simulink library "fast_library"  (Simulink 8.1)
settings: Solver=ode45  StartTime=0.0  StopTime=10.0  RelTol=1e-3
libraries: xbsIndex_r4 x439, casper_library_misc x3, xps_library x2
(part 1 of 3)
settings Model: Creator=zhuyan  LastModifiedBy=zhuyan

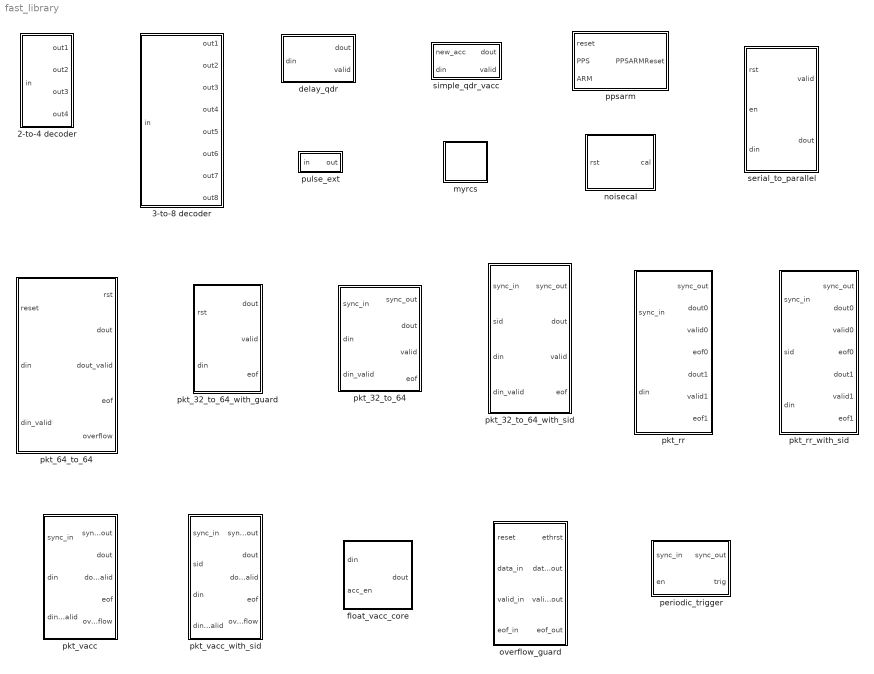
== system fast_library ==
  2-to-4 decoder : Subsystem  mask(decoder_2_4){}
      mask help: 2 to 4 decoder
  3-to-8 decoder : Subsystem  mask(decoder_3_8){}
      mask help: 3 to 8 decoder
  delay_qdr : Subsystem  mask(delay_qdr){DelayLen=1022, qdr_slot=qdr1}
      mask prompts: DelayLen "Delay Length (even number >=14):"; qdr_slot "QDR Slot:"
      mask init:
      | set_param([gcb, '/qdr'], 'which_qdr', qdr_slot);
      mask TypeOptions qdr_slot: qdr0 | qdr1 | qdr2 | qdr3
  float_vacc_core : Subsystem  mask(float_vacc_core){veclen=16, arith_type=1, conv_latency=3, add_latency=2, bram_latency=2, mux_latency=1}
      mask prompts: veclen "Vector Length"; arith_type "Arithmetic Type (0=Unsigned, 1=Signed)"; conv_latency "Convert Lantency"; add_latency "Add Latency"; bram_latency "BRAM Latency"; mux_latency "Mux Latency"
      mask help:
      | Currently only Signed arithmetic supported
      | acc_en = 0 --> Load a vector (start a new accumulation)
      | acc_en = 1 --> Accumulate
      mask init:
      | float_vacc_core_init(gcb, ...
      |     'veclen', veclen, ...
      |     'arith_type', arith_type, ...
      |     'conv_latency', conv_latency, ...
      |     'add_latency', add_latency, ...
      |     'bram_latency', bram_latency, ...
      |     'mux_latency', mux_latency);
  myrcs : Subsystem  mask(myrcs){proj_id=MYID}
      mask prompts: proj_id "Project ID:"
      mask help:
      | Revision control block.
      |
      | proj_id - exact 4 characters filled by user.
      | timestamp - seconds from unix epoch.
      | version - high 16 bits are major and low 16 bits are minor.
      |
      | The timestamp and version are taken from model properties.
      mask init:
      | blk = gcb();
      | sys = bdroot();
      | 
      | if length(proj_id) ~= 4
      |     error('Project ID must be exact 4 characters');
      | end
      | 
      | set_param(blk, 'LinkStatus', 'inactive')
      | 
      | rcs_id = proj_id(1)*256^3 + proj_id(2)*256^2 + proj_id(3)*256 + proj_id(4);
      | set_param([blk '/rcs_id'], 'const', num2str(rcs_id));
      | 
      | unix_epoch = datenum(1970, 1, 1, 0, 0, 0);
      | mdate = datenum(get_param(sys, 'LastModifiedDate'), 'ddd mmm dd HH:MM:SS yyyy');
      | unix_time = round((mdate - unix_epoch) * 24*60*60);
      | set_param([blk '/rcs_timestamp'], 'const', num2str(unix_time));
      | 
      | vers = sscanf(get_param(sys, 'ModelVersion'), '%d.%d');
      | rcs_ver = num2str(vers(1)*65536 + vers(2));
      | set_param([blk '/rcs_ver'], 'const', rcs_ver);
      mask Display: fprintf(proj_id);
  noisecal : Subsystem  mask(noisecal){}
      mask help:
      | Square wave to control external noise source.
      |
      | delay - number of clocks before the noise on signal after reset+latency
      | on - number of clocks in on state
      | off -number of clocks in off state
      |
      | sequence:
      | reset->delay->on->off->on->off->...
      mask Display:
      | port_label('input', 1, 'rst');
      | port_label('output', 1, 'cal');
      | disp('z^{-5}','texmode','on');
  overflow_guard : Subsystem  mask(overflow_guard){}
      mask help: Overflow gardian to ten_Gbe_v2 block
  periodic_trigger : Subsystem  mask(periodic_trigger){period=3}
  pkt_32_to_64 : Subsystem  mask(pkt_32_to_64){nbits=10}
      mask prompts: nbits "Packet Size in input length (2^?) :"
      mask help: packetizer 32-bits wide input into 64-bits wide packets and insert a 64-bit serial number at the packet head.
      mask init:
      | dstr = sprintf('packet length: %d bytes', 2^nbits * 4 + 8);
      | set_param(gcb, 'AttributesFormatString', dstr);
      settings: AttributesFormatString=packet length: 4104 bytes
      mask Display:
      | port_label('input', 1, 'sync_in');
      | port_label('input', 2, 'din');
      | port_label('input', 3, 'din_valid');
      | port_label('output', 1, 'sync_out');
      | port_label('output', 2, 'dout');
      | port_label('output', 3, 'valid');
      | port_label('output', 4, 'eof');
      | color('black');disp('z^{-3}','texmode','on');
  pkt_32_to_64_with_guard : Subsystem  mask(pkt_32_to_64_with_guard){nbits=10}
      mask prompts: nbits "Packet Size in input length (2^?) :"
      mask help:
      | valid data output 4 cycles later than reset signal.
      | serial number start from 1 (instead of 0) after reset signal.
      | Issue 10GbE block a reset signal before reset this block
      mask Display:
      | port_label('input', 1, 'rst');
      | port_label('input', 2, 'din');
      | port_label('output', 1, 'dout');
      | port_label('output', 2, 'valid');
      | port_label('output', 3, 'eof');
      | color('black');disp('z^{-4}','texmode','on');
      | fprintf('\n\n\n%dB', 2^nbits * 4 + 8);
  pkt_32_to_64_with_sid : Subsystem  mask(pkt_32_to_64_with_sid){nbits=10}
      mask prompts: nbits "Packet Size in input length (2^?) :"
      mask help: packetizer 32-bit wide input into 64-bit wide packets and insert a 64-bit header which consist of one 8-bit sid and one 56-bit serial number before sending out packet data.
      mask init:
      | dstr = sprintf('packet length: %d bytes', 2^nbits * 4 + 8);
      | set_param(gcb, 'AttributesFormatString', dstr);
      settings: AttributesFormatString=packet length: 4104 bytes
      mask Display:
      | port_label('input', 1, 'sync_in');
      | port_label('input', 2, 'sid');
      | port_label('input', 3, 'din');
      | port_label('input', 4, 'din_valid');
      | port_label('output', 1, 'sync_out');
      | port_label('output', 2, 'dout');
      | port_label('output', 3, 'valid');
      | port_label('output', 4, 'eof');
      | color('black');disp('z^{-3}','texmode','on');
  pkt_64_to_64 : Subsystem  mask{pktlen=1024, idlecycles=640, fifo_depth=2K}
      mask prompts: pktlen "Packet length in INPUT word (64bit):"; idlecycles "Idle cycles between packet:"; fifo_depth "FIFO depth (in 64bit word):"
      mask TypeOptions fifo_depth: 16 | 32 | 64 | 128 | 256 | 512 | 1K | 2K | 4K | 8K | 16K | 32K | 64K | 128K | 256K | 512K | 1M | 2M | 4M
  pkt_rr : Subsystem  mask(pkt_rr){nbits=9}
      mask prompts: nbits "Packet Size: (2^?)"
      mask help:
      | Split continous 64 bit input stream into packets and add one 64 bit serial number at each packet head.
      |
      | The output packets are placed into 2 output ports round robin, to match 2 10GbE yellow block.
      |
      | The packet size is counted in number of 64 bit (8 bytes) input word, the recommended packet size is 9 (4096 bytes).
  pkt_rr_with_sid : Subsystem  mask(pkt_rr_with_sid){nbits=9}
      mask prompts: nbits "Packet Size: (2^?)"
      mask help:
      | Split continous 64 bit input stream into packets and add one 64 bit serial number at each packet head.
      |
      | The output packets are placed into 2 output ports round robin, to match 2 10GbE yellow block.
      |
      | The packet size is counted in number of 64 bit (8 bytes) input word, the recommended packet size is 9 (4096 bytes).
  pkt_vacc : Subsystem  mask(pkt_vacc){spec_bits=8, pkt_bits=8, fifo_depth=16}
      mask prompts: spec_bits "Spectrum Size (2^?) in 64-bit word:"; pkt_bits "Packet Size (2^?):"; fifo_depth "FIFO Depth:"
      mask help:
      | For packetize bulk vacc output.
      |
      | 1. Split spectrum longer than 2^9 words (4k bytes) into 2^9 words packets.
      | 2. Leave spectrum shorter than 2^9 words as one single packet.
      | 3. Add a 64-bit serial number for each packet.
      mask init:
      | if spec_bits < pkt_bits
      |     error('Packet size should be equal or smaller than Spectrum size!');
      | elseif pkt_bits == spec_bits
      |     fifo_depth = '16';
      | elseif spec_bits > 20
      |     error('Spectrum size too large! should < 20');
      | else
      |     if spec_bits > 10
      |         fifo_depth = [num2str(2^(spec_bits - 11)) 'K'];
      |     else
      |         fifo_depth = num2str(2^(spec_bits - 1));
      |     end
      | end
      | 
      | % msgbox(fifo_depth);
      | %set_param([gcb '/FIFO'], 'depth', fifo_depth);
      | 
      | set_param(gcb, 'fifo_depth', fifo_depth);
  pkt_vacc_with_sid : Subsystem  mask(pkt_vacc_with_sid){spec_bits=8, pkt_bits=8, fifo_depth=16}
      mask prompts: spec_bits "Spectrum Size (2^?) in 64-bit word:"; pkt_bits "Packet Size (2^?):"; fifo_depth "FIFO Depth:"
      mask help:
      | For packetize bulk vacc output.
      |
      | 1. Split spectrum longer than 2^9 words (4k bytes) into 2^9 words packets.
      | 2. Leave spectrum shorter than 2^9 words as one single packet.
      | 3. Add a 64-bit serial number for each packet.
      mask init: same as fast_library/pkt_vacc
  ppsarm : Subsystem  mask(ppsarm){}
      mask help: PPS-ARM machanism
  pulse_ext : Subsystem  mask(pulse_ext){pulse_len=2}
      mask prompts: pulse_len "Length of Pulse"
      mask help: Extends a boolean signal to be high for the specified number of clocks after the last high input.
      mask init:
      | bits = ceil(log2(pulse_len+1));
      mask Help: eval('xlWeb(''http://casper.berkeley.edu/wiki/Pulse_ext'')')
  serial_to_parallel : Subsystem  mask(serial_to_parallel){n_elems=4}
      mask prompts: n_elems "Number of Parallel Elements:"
      mask init:
      | serial_to_parallel_init(gcb, ...
      |     'n_elems', n_elems)
  simple_qdr_vacc : Subsystem  mask(simple_qdr_vacc){vec_len=94, arith_type=Signed, n_bits=32, bin_pt=5, qdr_slot=qdr0}
      mask prompts: vec_len "Vector length (even number):"; arith_type "Output type:"; n_bits "Bit width (output):"; bin_pt "Binary point (output):"; qdr_slot "QDR slot:"
      mask help: It will output accumulated value from the 2nd new_acc
      mask init:
      | simple_qdr_vacc_init(gcb, ...
      |     'vec_len', vec_len, ...
      |     'arith_type', arith_type, ...
      |     'n_bits', n_bits, ...
      |     'bin_pt', bin_pt, ...
      |     'qdr_slot', qdr_slot);
      mask TypeOptions arith_type: Signed | Unsigned
      mask TypeOptions qdr_slot: qdr0 | qdr1 | qdr2 | qdr3

== system fast_library/2-to-4 decoder ==
  in : Inport
  Inverter : xbsIndex_r4/Inverter  en=off  latency=0  dbl_ovrd=off  block_type=inv
  Inverter1 : xbsIndex_r4/Inverter  en=off  latency=0  dbl_ovrd=off  block_type=inv
  Logical{,1..3} (4 alike) : xbsIndex_r4/Logical  logical_function=AND  inputs=2  en=off  latency=0  precision=Full  arith_type=Unsigned  n_bits=16  bin_pt=0  align_bp=on  dbl_ovrd=off  block_type=logical
  high bit : xbsIndex_r4/Slice  nbits=1  boolean_output=off  mode=Upper Bit Location + Width  bit1=0  base1=MSB of Input  bit0=0  base0=LSB of Input  dbl_ovrd=off  block_type=slice
  low bit : xbsIndex_r4/Slice  nbits=1  boolean_output=off  mode=Lower Bit Location + Width  bit1=0  base1=MSB of Input  bit0=0  base0=LSB of Input  dbl_ovrd=off  block_type=slice
  out1 : Outport
  out2 : Outport  Port=2
  out3 : Outport  Port=3
  out4 : Outport  Port=4
  wires:
  Logical2/1 -> out3/1
  Logical1/1 -> out2/1
  Logical/1 -> out1/1
  Inverter/1 -> Logical2/2, Logical/1
  high bit/1 -> Logical3/2, Logical2/1, Inverter1/1
  low bit/1 -> Logical3/1, Logical1/1, Inverter/1
  Logical3/1 -> out4/1
  Inverter1/1 -> Logical1/2, Logical/2
  in/1 -> low bit/1, high bit/1

== system fast_library/3-to-8 decoder ==
  in : Inport
  2-to-4 decoder : Subsystem
  2-to-4 decoder1 : Subsystem
  Inverter : xbsIndex_r4/Inverter  en=off  latency=0  dbl_ovrd=off  block_type=inv
  Slice : xbsIndex_r4/Slice  nbits=1  boolean_output=off  mode=Lower Bit Location + Width  bit1=0  base1=MSB of Input  bit0=1  base0=LSB of Input  dbl_ovrd=off  block_type=slice
  Slice1 : xbsIndex_r4/Slice  nbits=1  boolean_output=off  mode=Lower Bit Location + Width  bit1=0  base1=MSB of Input  bit0=0  base0=LSB of Input  dbl_ovrd=off  block_type=slice
  Slice2 : xbsIndex_r4/Slice  nbits=1  boolean_output=off  mode=Lower Bit Location + Width  bit1=0  base1=MSB of Input  bit0=2  base0=LSB of Input  dbl_ovrd=off  block_type=slice
  out1 : Outport
  out2 : Outport  Port=2
  out3 : Outport  Port=3
  out4 : Outport  Port=4
  out5 : Outport  Port=5
  out6 : Outport  Port=6
  out7 : Outport  Port=7
  out8 : Outport  Port=8
  wires:
  Slice2/1 -> 2-to-4 decoder1/3(EN), Inverter/1
  Slice1/1 -> 2-to-4 decoder1/1(A), 2-to-4 decoder/1(A)
  2-to-4 decoder1/4(D3) -> out8/1
  2-to-4 decoder/3(D2) -> out3/1
  2-to-4 decoder1/3(D2) -> out7/1
  2-to-4 decoder1/1(D0) -> out5/1
  2-to-4 decoder/4(D3) -> out4/1
  2-to-4 decoder/2(D1) -> out2/1
  2-to-4 decoder/1(D0) -> out1/1
  2-to-4 decoder1/2(D1) -> out6/1
  in/1 -> Slice1/1, Slice2/1, Slice/1
  Inverter/1 -> 2-to-4 decoder/3(EN)
  Slice/1 -> 2-to-4 decoder1/2(B), 2-to-4 decoder/2(B)

== system fast_library/delay_qdr ==
  din : Inport
  Constant3 : xbsIndex_r4/Constant  const=15  gui_display_data_type=Fixed-point  arith_type=Unsigned  n_bits=4  bin_pt=0  preci_type=Single  exp_width=8  frac_width=24  explicit_period=off  period=1  equ=P=C  opselect=C  inp2=PCIN>>17  opr=+  inp1=P  carry=CIN  dbl_ovrd=off  block_type=constant
  Constant4 : xbsIndex_r4/Constant  const=DelayLen-10-4  gui_display_data_type=Fixed-point  arith_type=Unsigned  n_bits=nextpow2(DelayLen)  bin_pt=0  preci_type=Single  exp_width=8  frac_width=24  explicit_period=on  period=1  equ=P=C  opselect=C  inp2=PCIN>>17  opr=+  inp1=P  carry=CIN  dbl_ovrd=off  block_type=constant
  Convert : xbsIndex_r4/Convert  gui_display_data_type=Fixed-point  arith_type=Unsigned  n_bits=36  bin_pt=0  float_type=Single  exp_bits=8  fraction_bits=24  quantization=Truncate  overflow=Wrap  en=off  latency=0  dbl_ovrd=off  pipeline=off  block_type=convert
      settings: block_version=11.4
  Delay : xbsIndex_r4/Delay  rst=off  infoeditControl=Selection of Reset will increase slice count due to use of real FFs and instead of SRLs  en=off  latency=1  dbl_ovrd=off  reg_retiming=off  block_type=delay
  Delay1 : xbsIndex_r4/Delay  rst=off  infoeditControl=Selection of Reset will increase slice count due to use of real FFs and instead of SRLs  en=off  latency=1  dbl_ovrd=off  reg_retiming=off  block_type=delay
  Delay2 : xbsIndex_r4/Delay  rst=off  infoeditControl=Selection of Reset will increase slice count due to use of real FFs and instead of SRLs  en=off  latency=1  dbl_ovrd=off  reg_retiming=off  block_type=delay
  Gateway Out{1..6} (6 alike) : xbsIndex_r4/Gateway Out  inherit_from_input=off  hdl_port=on  timing_constraint=None  locs_specified=off  LOCs={}  UseAsDAC=off  DACChannel='1'  block_type=gatewayout
  Inverter2 : xbsIndex_r4/Inverter  en=off  latency=0  dbl_ovrd=off  block_type=inv
  Mux3 : xbsIndex_r4/Mux  inputs=2  en=off  latency=0  precision=Full  arith_type="Signed  (2's comp)"  n_bits=8  bin_pt=2  quantization=Truncate  overflow=Wrap  dbl_ovrd=off  block_type=mux
      settings: xl_area=[0, 0, 0, 0, 0, 0, 0]
  Reinterpret : xbsIndex_r4/Reinterpret  force_arith_type=on  arith_type=Unsigned  force_bin_pt=on  bin_pt=0  block_type=reinterpret
  Relational : xbsIndex_r4/Relational  mode=a=b  en=off  latency=0  dbl_ovrd=off  block_type=relational
  Scope : Scope  NumInputPorts=6
      settings: YMin=-5~-5~-5~-5~-5~-5  YMax=5~5~5~5~5~5  SaveName=Scope
  Slice1 : xbsIndex_r4/Slice  nbits=1  boolean_output=off  mode=Two Bit Locations  bit1=0  base1=MSB of Input  bit0=1  base0=LSB of Input  dbl_ovrd=off  block_type=slice
  Slice2 : xbsIndex_r4/Slice  nbits=1  boolean_output=off  mode=Two Bit Locations  bit1=0  base1=MSB of Input  bit0=1  base0=LSB of Input  dbl_ovrd=off  block_type=slice
  Terminator : Terminator
  Terminator1 : Terminator
  Terminator2 : Terminator
  qdr : xps_library/qdr  Tag=xps:qdr  which_qdr=qdr1  qdr_awidth=12  use_sniffer=off
  rd/wr : xbsIndex_r4/Counter  cnt_type=Free Running  cnt_to=Inf  operation=Up  start_count=1  cnt_by_val=1  arith_type=Unsigned  n_bits=1  bin_pt=0  load_pin=off  rst=off  en=off  explicit_period=on  period=1  dbl_ovrd=off  use_behavioral_HDL=off  implementation=Fabric  block_type=counter
  rd_addr : xbsIndex_r4/Counter  cnt_type=Count Limited  cnt_to=DelayLen-1  operation=Up  start_count=0  cnt_by_val=1  arith_type=Unsigned  n_bits=nextpow2(DelayLen)  bin_pt=0  load_pin=off  rst=on  en=off  explicit_period=on  period=1  dbl_ovrd=off  use_behavioral_HDL=off  implementation=Fabric  use_rpm=off  block_type=counter
      settings: xl_area=[0, 0, 0, 0, 0, 0, 0]
  wr_addr : xbsIndex_r4/Counter  cnt_type=Count Limited  cnt_to=DelayLen-1  operation=Up  start_count=0  cnt_by_val=1  arith_type=Unsigned  n_bits=nextpow2(DelayLen)  bin_pt=0  load_pin=off  rst=off  en=off  explicit_period=on  period=1  dbl_ovrd=off  use_behavioral_HDL=off  implementation=Fabric  use_rpm=off  block_type=counter
      settings: xl_area=[0, 0, 0, 0, 0, 0, 0]
  dout : Outport
  valid : Outport  Port=2
  wires:
  Slice2/1 -> Mux3/3
  qdr/5 -> Terminator2/1
  Constant4/1 -> Relational/2
  Mux3/1 -> Gateway Out2/1, qdr/4
  Convert/1 -> Gateway Out3/1, qdr/5
  qdr/3 -> Terminator/1
  rd_addr/1 -> Slice1/1
  wr_addr/1 -> Relational/1, Slice2/1
  Delay/1 -> rd_addr/1
  Constant3/1 -> qdr/3
  qdr/4 -> Terminator1/1
  Relational/1 -> Delay/1
  Slice1/1 -> Mux3/2
  qdr/2 -> Delay2/1
  qdr/1 -> Delay1/1
  Gateway Out6/1 -> Scope/1
  Gateway Out1/1 -> Scope/2
  Gateway Out2/1 -> Scope/3
  Gateway Out3/1 -> Scope/4
  Gateway Out4/1 -> Scope/5
  Gateway Out5/1 -> Scope/6
  rd/wr/1 -> Gateway Out1/1, qdr/2, Inverter2/1, Mux3/1
  Inverter2/1 -> Gateway Out6/1, qdr/1
  Delay1/1 -> Gateway Out5/1, dout/1
  Delay2/1 -> Gateway Out4/1, valid/1
  din/1 -> Reinterpret/1
  Reinterpret/1 -> Convert/1

== system fast_library/float_vacc_core ==
  note: This BRAM and counter is exactly what is inside the green
      | Delay BRAM block. The functionality was extracted to avoid
      | library issues.
  din : Inport
  acc_en : Inport  Port=2
  Adder : xbsIndex_r4/AddSub  mode=Addition  use_carryin=off  use_carryout=off  en=off  latency=2  precision=Full  arith_type="Signed  (2's comp)"  n_bits=32  bin_pt=7  quantization=Truncate  overflow=Wrap  dbl_ovrd=off  use_behavioral_HDL=on  hw_selection=Fabric  pipelined=on  use_rpm=on  block_type=addsub
      settings: xl_area=[0, 0, 0, 0, 0, 0, 0]  block_version=10.1.2
  BRAM : xbsIndex_r4/Single Port RAM  depth=16  initVector=0  distributed_mem=Block RAM  write_mode=Read Before Write  rst=off  init_reg=0  en=off  latency=2  dbl_ovrd=off  optimize=Area  block_type=spram
      settings: xl_area=[0, 0, 0, 0, 0, 0, 0]  block_version=10.1.2
  Constant : xbsIndex_r4/Constant  const=0  gui_display_data_type=Floating-point  arith_type=Floating-point  n_bits=1  bin_pt=0  preci_type=Single  exp_width=8  frac_width=24  explicit_period=on  period=1  equ=P=C  opselect=C  inp2=PCIN>>17  opr=+  inp1=P  carry=CIN  dbl_ovrd=off  block_type=constant
      settings: block_version=10.1.2
  Constant2 : xbsIndex_r4/Constant  const=1  gui_display_data_type=Fixed-point  arith_type=Boolean  n_bits=1  bin_pt=0  preci_type=Single  exp_width=8  frac_width=24  explicit_period=on  period=1  equ=P=C  opselect=C  inp2=PCIN>>17  opr=+  inp1=P  carry=CIN  dbl_ovrd=off  block_type=constant
      settings: block_version=10.1.2
  Convert : xbsIndex_r4/Convert  gui_display_data_type=Floating-point  arith_type=Floating-point  n_bits=16  bin_pt=14  float_type=Single  exp_bits=8  fraction_bits=24  quantization=Truncate  overflow=Wrap  en=off  latency=3  dbl_ovrd=off  pipeline=on  block_type=convert
  Counter : xbsIndex_r4/Counter  cnt_type=Count Limited  cnt_to=7  operation=Up  start_count=0  cnt_by_val=1  arith_type=Unsigned  n_bits=4  bin_pt=0  load_pin=off  rst=off  en=off  explicit_period=off  period=1  dbl_ovrd=off  use_behavioral_HDL=off  implementation=Fabric  use_rpm=off  block_type=counter
      settings: xl_area=[0, 0, 0, 0, 0, 0, 0]  block_version=10.1.2
  Delay : xbsIndex_r4/Delay  rst=off  infoeditControl=Selection of Reset will increase slice count due to use of real FFs and instead of SRLs  en=off  latency=3  dbl_ovrd=off  reg_retiming=off  block_type=delay
  Delay1 : xbsIndex_r4/Delay  rst=off  infoeditControl=Selection of Reset will increase slice count due to use of real FFs and instead of SRLs  en=off  latency=3  dbl_ovrd=off  reg_retiming=off  block_type=delay
  Mux : xbsIndex_r4/Mux  inputs=2  en=off  latency=1  precision=Full  arith_type="Signed  (2's comp)"  n_bits=8  bin_pt=2  quantization=Truncate  overflow=Wrap  dbl_ovrd=off  block_type=mux
      settings: xl_area=[0, 0, 0, 0, 0, 0, 0]  block_version=10.1.2
  dout : Outport
  wires:
  acc_en/1 -> Delay/1
  Constant/1 -> Mux/2
  din/1 -> Convert/1
  Adder/1 -> dout/1, BRAM/2
  Counter/1 -> BRAM/1
  Constant2/1 -> BRAM/3
  Convert/1 -> Adder/1
  Delay/1 -> Mux/1
  Mux/1 -> Adder/2
  BRAM/1 -> Delay1/1
  Delay1/1 -> Mux/3

== system fast_library/myrcs ==
  id : Subsystem  Tag=xps:sw_reg  AncestorBlock=xps_library/software register  mask(swreg){io_dir=To Processor, io_delay=0, sample_period=1, names=reg, bitwidths=32, bin_pts=0, arith_types=0, sim_port=off, show_format=on}
      mask prompts: io_dir "I/O direction"; io_delay "I/O delay"; sample_period "Sample period"; names "Bitfield names [msb...lsb]"; bitwidths "Bitfield widths"; bin_pts "Bitfield binary pts"; arith_types "Bitfield types, ufix=0, fix=1, bool=2"; sim_port "Provide sim input/output?"; show_format "Print format string?"
      mask help: A 32-bit software-accessible register. Can be divided into bitfields of varying widths and types using the fields in the block mask.
      mask init:
      | swreg_init(gcb)
      settings: AttributesFormatString=1output:uf32.0
      mask TypeOptions io_dir: To Processor | From Processor
      mask Callback io_dir:
      | mask_enables = get_param(gcb, 'MaskEnables');
      | mask_names = get_param(gcb, 'MaskNames');
      | if strcmp(get_param(gcb, 'io_dir'), 'To Processor'),
      |     mask_enables{ismember(mask_names, 'sample_period')} = 'off';
      | else
      |     mask_enables{ismember(mask_names, 'sample_period')} = 'on';
      | end
      | set_param(gcb, 'MaskEnables', mask_enables);
  rcs_id : xbsIndex_r4/Constant  const=1297697092  gui_display_data_type=Fixed-point  arith_type=Unsigned  n_bits=32  bin_pt=0  preci_type=Single  exp_width=8  frac_width=24  explicit_period=on  period=1  equ=P=C  opselect=C  inp2=PCIN>>17  opr=+  inp1=P  carry=CIN  dbl_ovrd=off  block_type=constant
  rcs_timestamp : xbsIndex_r4/Constant  const=1550549974  gui_display_data_type=Fixed-point  arith_type=Unsigned  n_bits=32  bin_pt=0  preci_type=Single  exp_width=8  frac_width=24  explicit_period=on  period=1  equ=P=C  opselect=C  inp2=PCIN>>17  opr=+  inp1=P  carry=CIN  dbl_ovrd=off  block_type=constant
  rcs_ver : xbsIndex_r4/Constant  const=65582  gui_display_data_type=Fixed-point  arith_type=Unsigned  n_bits=32  bin_pt=0  preci_type=Single  exp_width=8  frac_width=24  explicit_period=on  period=1  equ=P=C  opselect=C  inp2=PCIN>>17  opr=+  inp1=P  carry=CIN  dbl_ovrd=off  block_type=constant
  timestamp : Subsystem  Tag=xps:sw_reg  AncestorBlock=xps_library/software register  mask(swreg){io_dir=To Processor, io_delay=0, sample_period=1, names=reg, bitwidths=32, bin_pts=0, arith_types=0, sim_port=off, show_format=on}
      mask prompts: io_dir "I/O direction"; io_delay "I/O delay"; sample_period "Sample period"; names "Bitfield names [msb...lsb]"; bitwidths "Bitfield widths"; bin_pts "Bitfield binary pts"; arith_types "Bitfield types, ufix=0, fix=1, bool=2"; sim_port "Provide sim input/output?"; show_format "Print format string?"
      mask help: A 32-bit software-accessible register. Can be divided into bitfields of varying widths and types using the fields in the block mask.
      mask init:
      | swreg_init(gcb)
      settings: AttributesFormatString=1output:uf32.0
      mask TypeOptions io_dir: To Processor | From Processor
      mask Callback io_dir:
      | mask_enables = get_param(gcb, 'MaskEnables');
      | mask_names = get_param(gcb, 'MaskNames');
      | if strcmp(get_param(gcb, 'io_dir'), 'To Processor'),
      |     mask_enables{ismember(mask_names, 'sample_period')} = 'off';
      | else
      |     mask_enables{ismember(mask_names, 'sample_period')} = 'on';
      | end
      | set_param(gcb, 'MaskEnables', mask_enables);
  ver : Subsystem  Tag=xps:sw_reg  AncestorBlock=xps_library/software register  mask(swreg){io_dir=To Processor, io_delay=0, sample_period=1, names=reg, bitwidths=32, bin_pts=0, arith_types=0, sim_port=off, show_format=on}
      mask prompts: io_dir "I/O direction"; io_delay "I/O delay"; sample_period "Sample period"; names "Bitfield names [msb...lsb]"; bitwidths "Bitfield widths"; bin_pts "Bitfield binary pts"; arith_types "Bitfield types, ufix=0, fix=1, bool=2"; sim_port "Provide sim input/output?"; show_format "Print format string?"
      mask help: A 32-bit software-accessible register. Can be divided into bitfields of varying widths and types using the fields in the block mask.
      mask init:
      | swreg_init(gcb)
      settings: AttributesFormatString=1output:uf32.0
      mask TypeOptions io_dir: To Processor | From Processor
      mask Callback io_dir:
      | mask_enables = get_param(gcb, 'MaskEnables');
      | mask_names = get_param(gcb, 'MaskNames');
      | if strcmp(get_param(gcb, 'io_dir'), 'To Processor'),
      |     mask_enables{ismember(mask_names, 'sample_period')} = 'off';
      | else
      |     mask_enables{ismember(mask_names, 'sample_period')} = 'on';
      | end
      | set_param(gcb, 'MaskEnables', mask_enables);
  wires:
  rcs_id/1 -> id/1(out_reg)
  rcs_ver/1 -> ver/1(out_reg)
  rcs_timestamp/1 -> timestamp/1(out_reg)

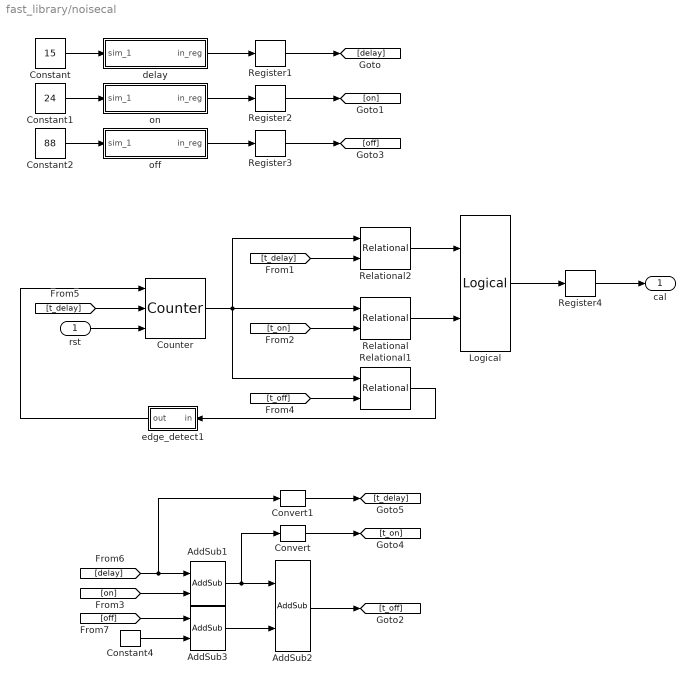
== system fast_library/noisecal ==
  rst : Inport
  AddSub1 : xbsIndex_r4/AddSub  mode=Addition  use_carryin=off  use_carryout=off  en=off  latency=2  precision=Full  arith_type=Unsigned  n_bits=32  bin_pt=0  quantization=Truncate  overflow=Wrap  dbl_ovrd=off  use_behavioral_HDL=on  hw_selection=Fabric  pipelined=off  block_type=addsub
  AddSub2 : xbsIndex_r4/AddSub  mode=Addition  use_carryin=off  use_carryout=off  en=off  latency=2  precision=Full  arith_type=Unsigned  n_bits=32  bin_pt=0  quantization=Truncate  overflow=Wrap  dbl_ovrd=off  use_behavioral_HDL=on  hw_selection=Fabric  pipelined=off  block_type=addsub
  AddSub3 : xbsIndex_r4/AddSub  mode=Subtraction  use_carryin=off  use_carryout=off  en=off  latency=2  precision=User Defined  arith_type=Unsigned  n_bits=33  bin_pt=0  quantization=Truncate  overflow=Wrap  dbl_ovrd=off  use_behavioral_HDL=on  hw_selection=Fabric  pipelined=off  block_type=addsub
  Constant : Constant  Value=15
  Constant1 : Constant  Value=24
  Constant2 : Constant  Value=88
  Constant4 : xbsIndex_r4/Constant  const=3  gui_display_data_type=Fixed-point  arith_type=Unsigned  n_bits=2  bin_pt=0  preci_type=Single  exp_width=8  frac_width=24  explicit_period=on  period=1  equ=P=C  opselect=C  inp2=PCIN>>17  opr=+  inp1=P  carry=CIN  dbl_ovrd=off  block_type=constant
  Convert : xbsIndex_r4/Convert  gui_display_data_type=Fixed-point  arith_type=Unsigned  n_bits=34  bin_pt=0  float_type=Single  exp_bits=8  fraction_bits=24  quantization=Truncate  overflow=Wrap  en=off  latency=2  dbl_ovrd=off  pipeline=off  block_type=convert
  Convert1 : xbsIndex_r4/Convert  gui_display_data_type=Fixed-point  arith_type=Unsigned  n_bits=34  bin_pt=0  float_type=Single  exp_bits=8  fraction_bits=24  quantization=Truncate  overflow=Wrap  en=off  latency=4  dbl_ovrd=off  pipeline=off  block_type=convert
  Counter : xbsIndex_r4/Counter  cnt_type=Free Running  cnt_to=Inf  operation=Up  start_count=0  cnt_by_val=1  arith_type=Unsigned  n_bits=34  bin_pt=0  load_pin=on  rst=on  en=off  explicit_period=on  period=1  dbl_ovrd=off  use_behavioral_HDL=on  implementation=Fabric  block_type=counter
  Logical : xbsIndex_r4/Logical  logical_function=XOR  inputs=2  en=off  latency=1  precision=Full  arith_type=Unsigned  n_bits=16  bin_pt=0  align_bp=on  dbl_ovrd=off  block_type=logical
  Register{1..4} (4 alike) : xbsIndex_r4/Register  init=0  rst=off  en=off  dbl_ovrd=off  block_type=register
  Relational : xbsIndex_r4/Relational  mode=a<b  en=off  latency=2  dbl_ovrd=off  block_type=relational
  Relational1 : xbsIndex_r4/Relational  mode=a<b  en=off  latency=2  dbl_ovrd=off  block_type=relational
  Relational2 : xbsIndex_r4/Relational  mode=a<b  en=off  latency=2  dbl_ovrd=off  block_type=relational
  delay : Subsystem  Tag=xps:sw_reg  AncestorBlock=xps_library/software register  mask(swreg){io_dir=From Processor, io_delay=0, sample_period=1, names=reg, bitwidths=32, bin_pts=0, arith_types=0, sim_port=on, show_format=off}
      mask prompts: io_dir "I/O direction"; io_delay "I/O delay"; sample_period "Sample period"; names "Bitfield names [msb...lsb]"; bitwidths "Bitfield widths"; bin_pts "Bitfield binary pts"; arith_types "Bitfield types, ufix=0, fix=1, bool=2"; sim_port "Provide sim input/output?"; show_format "Print format string?"
      mask help: A 32-bit software-accessible register. Can be divided into bitfields of varying widths and types using the fields in the block mask.
      mask init:
      | swreg_init(gcb)
      settings: AttributesFormatString=1input
      mask TypeOptions io_dir: To Processor | From Processor
      mask Callback io_dir:
      | mask_enables = get_param(gcb, 'MaskEnables');
      | mask_names = get_param(gcb, 'MaskNames');
      | if strcmp(get_param(gcb, 'io_dir'), 'To Processor'),
      |     mask_enables{ismember(mask_names, 'sample_period')} = 'off';
      | else
      |     mask_enables{ismember(mask_names, 'sample_period')} = 'on';
      | end
      | set_param(gcb, 'MaskEnables', mask_enables);
  edge_detect1 : Subsystem  AncestorBlock=casper_library_misc/edge_detect  mask(edge_detect){edge=Falling, polarity=Active High, x_in=[0 0.08 0.08 0.16 0.16 0.24 0.24 0.32 0.32 0.4], y_in=[-1 -1  1  1  1  1  1  1  1  1], x_out=[0.6 0.68 0.68 0.76 0.76 0.84 0.84 0.92 0.92 1], y_out=[-1 -1  1  1 -1 -1 -1 -1 -1 -1]}
      mask prompts: edge "Edge Type"; polarity "Output Polarity"; x_in "Input X Positions"; y_in "Input Y Positions"; x_out "Output X Positions"; y_out "Output Y Positions"
      mask help: Output is active for one-cycle after each edge of the specified type (i.e. rising, falling or both).
      mask init:
      | edge_detect_init(gcb,...
      |     'edge',edge,...
      |     'polarity',polarity,...
      |     'x_in',x_in,...
      |     'x_out',x_out,...
      |     'y_in',y_in,...
      |     'y_out',y_out);
      | 
      | x_in_num=str2num(getfield(getfield(get_param(gcb,'UserData'),'parameters'),'x_in'));
      | x_out_num=str2num(getfield(getfield(get_param(gcb,'UserData'),'parameters'),'x_out'));
      | y_in_num=str2num(getfield(getfield(get_param(gcb,'UserData'),'parameters'),'y_in'));
      | y_out_num=str2num(getfield(getfield(get_param(gcb,'UserData'),'parameters'),'y_out'));
      settings: AttributesFormatString=|
      | falling edges
      | active high
      mask Help: Output is active for one-cycle after each edge of the specified type (i.e. rising, falling, or both).  Latency is zero.
      mask TypeOptions edge: Rising | Falling | Both
      mask TypeOptions polarity: Active High | Active Low
      mask Display:
      | plot(x_in_num,0.5+y_in_num*0.2);
      | plot(x_out_num,0.5+y_out_num*0.2);
  off : Subsystem  Tag=xps:sw_reg  AncestorBlock=xps_library/software register  mask(swreg){io_dir=From Processor, io_delay=0, sample_period=1, names=reg, bitwidths=32, bin_pts=0, arith_types=0, sim_port=on, show_format=off}
      mask prompts: io_dir "I/O direction"; io_delay "I/O delay"; sample_period "Sample period"; names "Bitfield names [msb...lsb]"; bitwidths "Bitfield widths"; bin_pts "Bitfield binary pts"; arith_types "Bitfield types, ufix=0, fix=1, bool=2"; sim_port "Provide sim input/output?"; show_format "Print format string?"
      mask help: A 32-bit software-accessible register. Can be divided into bitfields of varying widths and types using the fields in the block mask.
      mask init:
      | swreg_init(gcb)
      settings: AttributesFormatString=1input
      mask TypeOptions io_dir: To Processor | From Processor
      mask Callback io_dir:
      | mask_enables = get_param(gcb, 'MaskEnables');
      | mask_names = get_param(gcb, 'MaskNames');
      | if strcmp(get_param(gcb, 'io_dir'), 'To Processor'),
      |     mask_enables{ismember(mask_names, 'sample_period')} = 'off';
      | else
      |     mask_enables{ismember(mask_names, 'sample_period')} = 'on';
      | end
      | set_param(gcb, 'MaskEnables', mask_enables);
  on : Subsystem  Tag=xps:sw_reg  AncestorBlock=xps_library/software register  mask(swreg){io_dir=From Processor, io_delay=0, sample_period=1, names=reg, bitwidths=32, bin_pts=0, arith_types=0, sim_port=on, show_format=off}
      mask prompts: io_dir "I/O direction"; io_delay "I/O delay"; sample_period "Sample period"; names "Bitfield names [msb...lsb]"; bitwidths "Bitfield widths"; bin_pts "Bitfield binary pts"; arith_types "Bitfield types, ufix=0, fix=1, bool=2"; sim_port "Provide sim input/output?"; show_format "Print format string?"
      mask help: A 32-bit software-accessible register. Can be divided into bitfields of varying widths and types using the fields in the block mask.
      mask init:
      | swreg_init(gcb)
      settings: AttributesFormatString=1input
      mask TypeOptions io_dir: To Processor | From Processor
      mask Callback io_dir:
      | mask_enables = get_param(gcb, 'MaskEnables');
      | mask_names = get_param(gcb, 'MaskNames');
      | if strcmp(get_param(gcb, 'io_dir'), 'To Processor'),
      |     mask_enables{ismember(mask_names, 'sample_period')} = 'off';
      | else
      |     mask_enables{ismember(mask_names, 'sample_period')} = 'on';
      | end
      | set_param(gcb, 'MaskEnables', mask_enables);
  cal : Outport
  wires:
  Convert1/1 -> [t_delay]
  Convert/1 -> [t_on]
  [t_off] -> Relational1/2
  AddSub2/1 -> [t_off]
  AddSub3/1 -> AddSub2/2
  Constant4/1 -> AddSub3/2
  [off] -> AddSub3/1
  AddSub1/1 -> AddSub2/1, Convert/1
  [on] -> AddSub1/2
  [delay] -> AddSub1/1, Convert1/1
  Register4/1 -> cal/1
  Relational1/1 -> edge_detect1/1(in)
  delay/1(in_reg) -> Register1/1
  Constant2/1 -> off/1(sim_1)
  Constant1/1 -> on/1(sim_1)
  Register1/1 -> [delay]
  [t_on] -> Relational/2
  Counter/1 -> Relational/1, Relational2/1, Relational1/1
  [t_delay] -> Counter/2
  rst/1 -> Counter/3
  Register2/1 -> [on]
  off/1(in_reg) -> Register3/1
  Relational2/1 -> Logical/1
  edge_detect1/1(out) -> Counter/1
  Relational/1 -> Logical/2
  Register3/1 -> [off]
  on/1(in_reg) -> Register2/1
  Constant/1 -> delay/1(sim_1)
  Logical/1 -> Register4/1
  [t_delay] -> Relational2/2

== system fast_library/overflow_guard ==
  note: 3 extra delay to satisfy ten_gbe block reset logic
  reset : Inport
  data_in : Inport  Port=2
  valid_in : Inport  Port=3
  eof_in : Inport  Port=4
  Constant11 : xbsIndex_r4/Constant  const=1  gui_display_data_type=Boolean  arith_type=Boolean  n_bits=1  bin_pt=0  preci_type=Single  exp_width=8  frac_width=24  explicit_period=on  period=1  equ=P=C  opselect=C  inp2=PCIN>>17  opr=+  inp1=P  carry=CIN  dbl_ovrd=off  block_type=constant
  Constant3 : xbsIndex_r4/Constant  const=1  gui_display_data_type=Boolean  arith_type=Boolean  n_bits=32  bin_pt=0  preci_type=Single  exp_width=8  frac_width=24  explicit_period=on  period=1  equ=P=C  opselect=C  inp2=PCIN>>17  opr=+  inp1=P  carry=CIN  dbl_ovrd=off  block_type=constant
  Delay{1..4} (4 alike) : xbsIndex_r4/Delay  rst=off  infoeditControl=Selection of Reset will increase slice count due to use of real FFs and instead of SRLs  en=off  latency=1  dbl_ovrd=off  reg_retiming=off  block_type=delay
  Delay5 : xbsIndex_r4/Delay  rst=off  infoeditControl=Selection of Reset will increase slice count due to use of real FFs and instead of SRLs  en=off  latency=4  dbl_ovrd=off  reg_retiming=off  block_type=delay
  Delay6 : xbsIndex_r4/Delay  rst=off  infoeditControl=Selection of Reset will increase slice count due to use of real FFs and instead of SRLs  en=off  latency=4  dbl_ovrd=off  reg_retiming=off  block_type=delay
  Delay8 : xbsIndex_r4/Delay  rst=off  infoeditControl=Selection of Reset will increase slice count due to use of real FFs and instead of SRLs  en=off  latency=4  dbl_ovrd=off  reg_retiming=off  block_type=delay
  Logical : xbsIndex_r4/Logical  logical_function=OR  inputs=2  en=off  latency=0  precision=Full  arith_type=Unsigned  n_bits=16  bin_pt=0  align_bp=on  dbl_ovrd=off  block_type=logical
  Logical1 : xbsIndex_r4/Logical  logical_function=OR  inputs=2  en=off  latency=0  precision=Full  arith_type=Unsigned  n_bits=16  bin_pt=0  align_bp=on  dbl_ovrd=off  block_type=logical
  Logical2 : xbsIndex_r4/Logical  logical_function=AND  inputs=2  en=off  latency=0  precision=Full  arith_type=Unsigned  n_bits=16  bin_pt=0  align_bp=on  dbl_ovrd=off  block_type=logical
  Logical3 : xbsIndex_r4/Logical  logical_function=AND  inputs=2  en=off  latency=0  precision=Full  arith_type=Unsigned  n_bits=16  bin_pt=0  align_bp=on  dbl_ovrd=off  block_type=logical
  Mux : xbsIndex_r4/Mux  inputs=2  en=off  latency=0  precision=Full  arith_type=Unsigned  n_bits=16  bin_pt=14  quantization=Truncate  overflow=Wrap  dbl_ovrd=off  block_type=mux
  Mux1 : xbsIndex_r4/Mux  inputs=2  en=off  latency=0  precision=Full  arith_type=Unsigned  n_bits=16  bin_pt=14  quantization=Truncate  overflow=Wrap  dbl_ovrd=off  block_type=mux
  edge_detect : casper_library_misc/edge_detect  edge=Rising  polarity=Active High  x_in=[0 0.08 0.08 0.16 0.16 0.24 0.24 0.32 0.32 0.4]  y_in="[-1 -1  1  1  1  1  1  1  1  1]"  x_out=[0.6 0.68 0.68 0.76 0.76 0.84 0.84 0.92 0.92 1]  y_out="[-1 -1  1  1 -1 -1 -1 -1 -1 -1]"
  eth_on : xbsIndex_r4/Register  init=0  rst=off  en=on  dbl_ovrd=off  block_type=register
  in_transmisson : xbsIndex_r4/Register  init=0  rst=on  en=on  dbl_ovrd=off  block_type=register
  ethrst : Outport
  data_out : Outport  Port=2
  valid_out : Outport  Port=3
  eof_out : Outport  Port=4
  wires:
  Delay4/1 -> Mux1/2, Logical1/1
  Delay1/1 -> Mux/2, Logical/1
  eof_in/1 -> Delay4/1, in_transmisson/2
  reset/1 -> eth_on/2, Delay3/1
  data_in/1 -> Delay2/1
  in_transmisson/1 -> Logical/2, Logical1/2
  valid_in/1 -> Delay1/1, in_transmisson/3
  Constant11/1 -> in_transmisson/1
  Mux/1 -> Logical2/2
  Mux1/1 -> Logical3/2
  Logical1/1 -> Mux1/3
  Logical/1 -> Mux/3
  Delay3/1 -> Mux1/1, Mux/1
  Logical2/1 -> Delay5/1
  Logical3/1 -> Delay6/1
  Delay2/1 -> Delay8/1
  eth_on/1 -> edge_detect/1, Logical3/1, Logical2/1
  Constant3/1 -> eth_on/1
  edge_detect/1 -> ethrst/1
  Delay5/1 -> valid_out/1
  Delay6/1 -> eof_out/1
  Delay8/1 -> data_out/1

== system fast_library/periodic_trigger ==
  sync_in : Inport
  en : Inport  Port=2
  Constant : xbsIndex_r4/Constant  const=period  gui_display_data_type=Fixed-point  arith_type=Unsigned  n_bits=nextpow2(period)  bin_pt=0  preci_type=Single  exp_width=8  frac_width=24  explicit_period=on  period=1  equ=P=C  opselect=C  inp2=PCIN>>17  opr=+  inp1=P  carry=CIN  dbl_ovrd=off  block_type=constant
  Counter : xbsIndex_r4/Counter  cnt_type=Free Running  cnt_to=8  operation=Up  start_count=0  cnt_by_val=1  arith_type=Unsigned  n_bits=nextpow2(period)  bin_pt=0  load_pin=off  rst=on  en=on  explicit_period=on  period=1  dbl_ovrd=off  use_behavioral_HDL=off  implementation=Fabric  block_type=counter
  Delay1 : xbsIndex_r4/Delay  rst=off  infoeditControl=Selection of Reset will increase slice count due to use of real FFs and instead of SRLs  en=off  latency=1  dbl_ovrd=off  reg_retiming=off  block_type=delay
  Delay2 : xbsIndex_r4/Delay  rst=off  infoeditControl=Selection of Reset will increase slice count due to use of real FFs and instead of SRLs  en=off  latency=1  dbl_ovrd=off  reg_retiming=off  block_type=delay
  Delay3 : xbsIndex_r4/Delay  rst=off  infoeditControl=Selection of Reset will increase slice count due to use of real FFs and instead of SRLs  en=off  latency=1  dbl_ovrd=off  reg_retiming=off  block_type=delay
  Logical : xbsIndex_r4/Logical  logical_function=OR  inputs=2  en=off  latency=0  precision=Full  arith_type=Unsigned  n_bits=16  bin_pt=0  align_bp=on  dbl_ovrd=off  block_type=logical
  Relational1 : xbsIndex_r4/Relational  mode=a=b  en=off  latency=0  dbl_ovrd=off  block_type=relational
  sync_out : Outport
  trig : Outport  Port=2
  wires:
  Delay1/1 -> sync_out/1
  Delay2/1 -> Delay1/1
  Delay3/1 -> trig/1
  sync_in/1 -> Logical/2, Delay2/1
  Constant/1 -> Relational1/1
  en/1 -> Counter/2
  Counter/1 -> Relational1/2
  Logical/1 -> Counter/1
  Relational1/1 -> Logical/1, Delay3/1

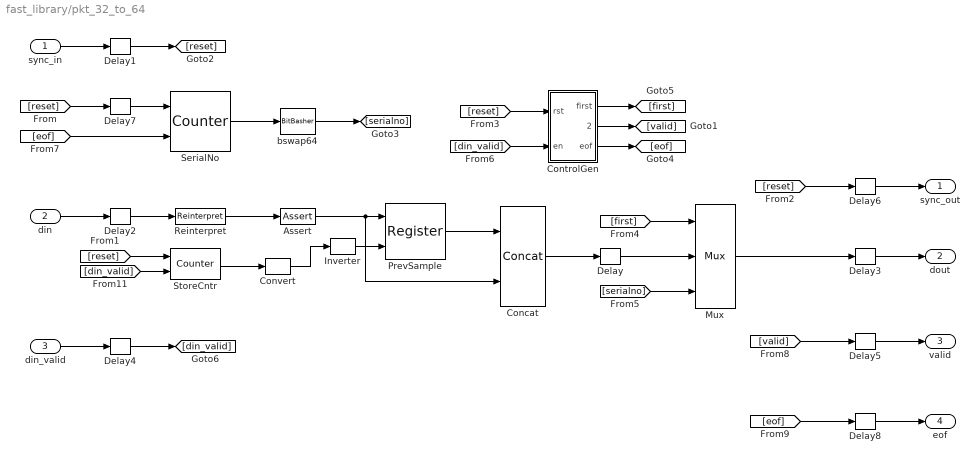
== system fast_library/pkt_32_to_64 ==
  sync_in : Inport
  din : Inport  Port=2
  din_valid : Inport  Port=3
  Assert : xbsIndex_r4/Assert  assert_type=on  type_source=Explicitly  gui_display_data_type=Fixed-point  arith_type=Unsigned  n_bits=32  bin_pt=0  preci_type=Single  exp_width=8  frac_width=24  assert_rate=off  rate_source=Explicitly  period=1  output_port=on  block_type=assert
  Concat : xbsIndex_r4/Concat  num_inputs=2  dbl_ovrd=off  block_type=concat
  ControlGen : Subsystem
  Convert : xbsIndex_r4/Convert  gui_display_data_type=Boolean  arith_type=Boolean  n_bits=16  bin_pt=14  float_type=Single  exp_bits=8  fraction_bits=24  quantization=Truncate  overflow=Wrap  en=off  latency=0  dbl_ovrd=off  pipeline=off  block_type=convert
  Delay{,1..5,7..8} (8 alike) : xbsIndex_r4/Delay  rst=off  infoeditControl=Selection of Reset will increase slice count due to use of real FFs and instead of SRLs  en=off  latency=1  dbl_ovrd=off  reg_retiming=off  block_type=delay
  Delay6 : xbsIndex_r4/Delay  rst=off  infoeditControl=Selection of Reset will increase slice count due to use of real FFs and instead of SRLs  en=off  latency=2  dbl_ovrd=off  reg_retiming=off  block_type=delay
  Inverter : xbsIndex_r4/Inverter  en=off  latency=0  dbl_ovrd=off  block_type=inv
  Mux : xbsIndex_r4/Mux  inputs=2  en=off  latency=0  precision=Full  arith_type=Unsigned  n_bits=16  bin_pt=14  quantization=Truncate  overflow=Wrap  dbl_ovrd=off  block_type=mux
  PrevSample : xbsIndex_r4/Register  init=0  rst=off  en=on  dbl_ovrd=off  block_type=register
  Reinterpret : xbsIndex_r4/Reinterpret  force_arith_type=on  arith_type=Unsigned  force_bin_pt=on  bin_pt=0  block_type=reinterpret
  SerialNo : xbsIndex_r4/Counter  cnt_type=Free Running  cnt_to=Inf  operation=Up  start_count=0  cnt_by_val=1  arith_type=Unsigned  n_bits=64  bin_pt=0  load_pin=off  rst=on  en=on  explicit_period=on  period=1  dbl_ovrd=off  use_behavioral_HDL=on  implementation=Fabric  block_type=counter
  StoreCntr : xbsIndex_r4/Counter  cnt_type=Free Running  cnt_to=Inf  operation=Up  start_count=0  cnt_by_val=1  arith_type=Unsigned  n_bits=1  bin_pt=0  load_pin=off  rst=on  en=on  explicit_period=on  period=1  dbl_ovrd=off  use_behavioral_HDL=off  implementation=Fabric  block_type=counter
  bswap64 : xbsIndex_r4/BitBasher  bitexpr=|  display_expr=off  sr_1=1  arith_type1=Unsigned  bin_pt1=0  sr_2=2  arith_type2=Unsigned  bin_pt2=0  sr_3=3  arith_type3=Unsigned  bin_pt3=0  sr_4=4  arith_type4=Unsigned  bin_pt4=0  dbl_ovrd=off  block_type=bitbasher
      | <!DOCTYPE HTML PUBLIC "-//W3C//DTD HTML 4.0//EN" "http://www.w3.org/TR/REC-html40/strict.dtd">
      | <html><head><meta name="qrichtext" content="1" /><style type="text/css">
      | p, li { white-space: pre-wrap; }
      | </style></head><body style=" font-family:'Segoe UI'; font-size:9pt; font-weight:400; font-style:normal;">
      | <p style=" margin-top:12px; margin-bottom:12px; margin-left:0px; margin-right:0px; -qt-block-indent:0; text-indent:0px;"><span style=" font-family:'MS Shell Dlg'; font-size:8pt;">b={a[7:0],a[15:8],a[23:16],a[31:24],a[39:32],a[47:40],a[55:48],a[63:56]}</span></p></body></html>
  sync_out : Outport
  dout : Outport  Port=2
  valid : Outport  Port=3
  eof : Outport  Port=4
  wires:
  ControlGen/3(eof) -> [eof]
  Convert/1 -> Inverter/1
  StoreCntr/1 -> Convert/1
  Inverter/1 -> PrevSample/2
  Concat/1 -> Delay/1
  [serialno] -> Mux/3
  PrevSample/1 -> Concat/1
  [reset] -> Delay7/1
  SerialNo/1 -> bswap64/1
  Delay/1 -> Mux/2
  din/1 -> Delay2/1
  [din_valid] -> ControlGen/2(en)
  [reset] -> ControlGen/1(rst)
  ControlGen/2(valid) -> [valid]
  sync_in/1 -> Delay1/1
  [reset] -> StoreCntr/1
  Reinterpret/1 -> Assert/1
  Assert/1 -> Concat/2, PrevSample/1
  Delay1/1 -> [reset]
  Delay2/1 -> Reinterpret/1
  Delay3/1 -> dout/1
  Mux/1 -> Delay3/1
  [reset] -> Delay6/1
  Delay6/1 -> sync_out/1
  [eof] -> SerialNo/2
  ControlGen/1(first) -> [first]
  [first] -> Mux/1
  Delay7/1 -> SerialNo/1
  din_valid/1 -> Delay4/1
  Delay4/1 -> [din_valid]
  [din_valid] -> StoreCntr/2
  Delay5/1 -> valid/1
  [valid] -> Delay5/1
  Delay8/1 -> eof/1
  [eof] -> Delay8/1
  bswap64/1 -> [serialno]

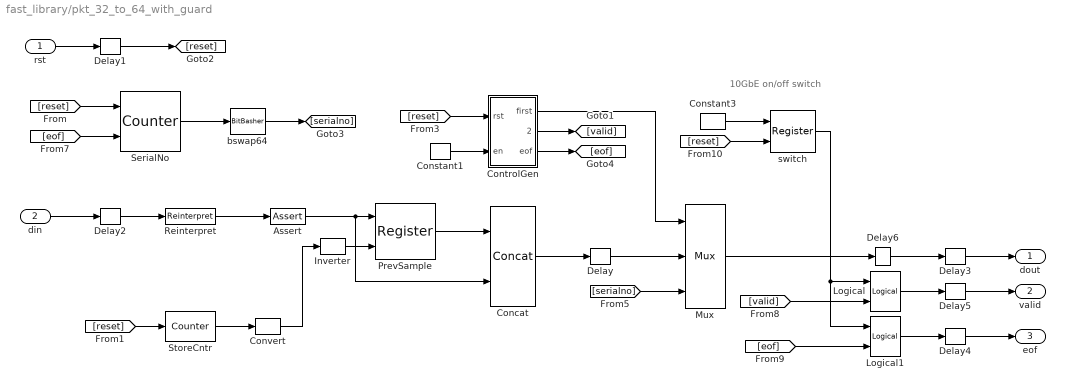
== system fast_library/pkt_32_to_64_with_guard ==
  note: 10GbE on/off switch
  rst : Inport
  din : Inport  Port=2
  Assert : xbsIndex_r4/Assert  assert_type=on  type_source=Explicitly  gui_display_data_type=Fixed-point  arith_type=Unsigned  n_bits=32  bin_pt=0  preci_type=Single  exp_width=8  frac_width=24  assert_rate=off  rate_source=Explicitly  period=1  output_port=on  block_type=assert
  Concat : xbsIndex_r4/Concat  num_inputs=2  dbl_ovrd=off  block_type=concat
  Constant1 : xbsIndex_r4/Constant  const=1  gui_display_data_type=Boolean  arith_type=Boolean  n_bits=16  bin_pt=14  preci_type=Single  exp_width=8  frac_width=24  explicit_period=on  period=1  equ=P=C  opselect=C  inp2=PCIN>>17  opr=+  inp1=P  carry=CIN  dbl_ovrd=off  block_type=constant
  Constant3 : xbsIndex_r4/Constant  const=1  gui_display_data_type=Boolean  arith_type=Boolean  n_bits=32  bin_pt=0  preci_type=Single  exp_width=8  frac_width=24  explicit_period=on  period=1  equ=P=C  opselect=C  inp2=PCIN>>17  opr=+  inp1=P  carry=CIN  dbl_ovrd=off  block_type=constant
  ControlGen : Subsystem
  Convert : xbsIndex_r4/Convert  gui_display_data_type=Boolean  arith_type=Boolean  n_bits=16  bin_pt=14  float_type=Single  exp_bits=8  fraction_bits=24  quantization=Truncate  overflow=Wrap  en=off  latency=0  dbl_ovrd=off  pipeline=off  block_type=convert
  Delay{,1..6} (7 alike) : xbsIndex_r4/Delay  rst=off  infoeditControl=Selection of Reset will increase slice count due to use of real FFs and instead of SRLs  en=off  latency=1  dbl_ovrd=off  reg_retiming=off  block_type=delay
  Inverter : xbsIndex_r4/Inverter  en=off  latency=0  dbl_ovrd=off  block_type=inv
  Logical : xbsIndex_r4/Logical  logical_function=AND  inputs=2  en=off  latency=1  precision=Full  arith_type=Unsigned  n_bits=16  bin_pt=0  align_bp=on  dbl_ovrd=off  block_type=logical
  Logical1 : xbsIndex_r4/Logical  logical_function=AND  inputs=2  en=off  latency=1  precision=Full  arith_type=Unsigned  n_bits=16  bin_pt=0  align_bp=on  dbl_ovrd=off  block_type=logical
  Mux : xbsIndex_r4/Mux  inputs=2  en=off  latency=0  precision=Full  arith_type=Unsigned  n_bits=16  bin_pt=14  quantization=Truncate  overflow=Wrap  dbl_ovrd=off  block_type=mux
  PrevSample : xbsIndex_r4/Register  init=0  rst=off  en=on  dbl_ovrd=off  block_type=register
  Reinterpret : xbsIndex_r4/Reinterpret  force_arith_type=on  arith_type=Unsigned  force_bin_pt=on  bin_pt=0  block_type=reinterpret
  SerialNo : xbsIndex_r4/Counter  cnt_type=Free Running  cnt_to=Inf  operation=Up  start_count=0  cnt_by_val=1  arith_type=Unsigned  n_bits=64  bin_pt=0  load_pin=off  rst=on  en=on  explicit_period=on  period=1  dbl_ovrd=off  use_behavioral_HDL=off  implementation=Fabric  block_type=counter
  StoreCntr : xbsIndex_r4/Counter  cnt_type=Free Running  cnt_to=Inf  operation=Up  start_count=0  cnt_by_val=1  arith_type=Unsigned  n_bits=1  bin_pt=0  load_pin=off  rst=on  en=off  explicit_period=on  period=1  dbl_ovrd=off  use_behavioral_HDL=off  implementation=Fabric  block_type=counter
  bswap64 : xbsIndex_r4/BitBasher  bitexpr=|  display_expr=off  sr_1=1  arith_type1=Unsigned  bin_pt1=0  sr_2=2  arith_type2=Unsigned  bin_pt2=0  sr_3=3  arith_type3=Unsigned  bin_pt3=0  sr_4=4  arith_type4=Unsigned  bin_pt4=0  dbl_ovrd=off  block_type=bitbasher
      | <!DOCTYPE HTML PUBLIC "-//W3C//DTD HTML 4.0//EN" "http://www.w3.org/TR/REC-html40/strict.dtd">
      | <html><head><meta name="qrichtext" content="1" /><style type="text/css">
      | p, li { white-space: pre-wrap; }
      | </style></head><body style=" font-family:'Segoe UI'; font-size:9pt; font-weight:400; font-style:normal;">
      | <p style=" margin-top:12px; margin-bottom:12px; margin-left:0px; margin-right:0px; -qt-block-indent:0; text-indent:0px;"><span style=" font-family:'MS Shell Dlg'; font-size:8pt;">b={a[7:0],a[15:8],a[23:16],a[31:24],a[39:32],a[47:40],a[55:48],a[63:56]}</span></p></body></html>
  switch : xbsIndex_r4/Register  init=0  rst=off  en=on  dbl_ovrd=off  block_type=register
  dout : Outport
  valid : Outport  Port=2
  eof : Outport  Port=3
  wires:
  ControlGen/3(eof) -> [eof]
  Convert/1 -> Inverter/1
  StoreCntr/1 -> Convert/1
  [eof] -> SerialNo/2
  Inverter/1 -> PrevSample/2
  Concat/1 -> Delay/1
  [serialno] -> Mux/3
  PrevSample/1 -> Concat/1
  [reset] -> SerialNo/1
  SerialNo/1 -> bswap64/1
  Delay/1 -> Mux/2
  ControlGen/1(first) -> Mux/1
  din/1 -> Delay2/1
  Constant1/1 -> ControlGen/2(en)
  [reset] -> ControlGen/1(rst)
  ControlGen/2(valid) -> [valid]
  rst/1 -> Delay1/1
  [reset] -> StoreCntr/1
  Reinterpret/1 -> Assert/1
  Assert/1 -> Concat/2, PrevSample/1
  Delay1/1 -> [reset]
  Delay2/1 -> Reinterpret/1
  Delay3/1 -> dout/1
  Delay4/1 -> eof/1
  Delay5/1 -> valid/1
  Mux/1 -> Delay6/1
  Constant3/1 -> switch/1
  [eof] -> Logical1/2
  [valid] -> Logical/2
  switch/1 -> Logical/1, Logical1/1
  [reset] -> switch/2
  Delay6/1 -> Delay3/1
  Logical/1 -> Delay5/1
  Logical1/1 -> Delay4/1
  bswap64/1 -> [serialno]
